simulink model "furutapendulumsim2"  (R2018a)
settings: Solver=VariableStepAuto  StartTime=0.0  StopTime=15  RelTol=1e-3
values from neighbouring files (symbols this model uses):
  A = [0,1,0,0 ... (first row only)    [furutapendulum.m]    (also in furutapendulum2.m = double(A); furutapendulum3.m = double(A); furutapendulum3_.m = double(A); furutapendulum4.m = double(A))
  B = [0 ... (first row only)    [furutapendulum.m]    (also in furutapendulum2.m = double(B); furutapendulum3.m = double(B); furutapendulum3_.m = double(B); furutapendulum4.m = double(B))
  length_base = 10e-3    (= 0.01)    [furutapendulum2.m]    (also in furutapendulum3.m; furutapendulum4.m)
  length_vert_cylinder = 200e-3    (= 0.2)    [furutapendulum2.m]    (also in furutapendulum3.m; furutapendulum4.m)
  m = 3.3e-3    (= 0.0033)    [furutapendulum2.m]    (also in furutapendulum3.m; furutapendulum4.m)
  radius_vert_cylinder = 10e-3    (= 0.01)    [furutapendulum2.m]    (also in furutapendulum3.m; furutapendulum4.m)
  s = tf('s')    [furutapendulum2.m]    (also in furutapendulum3.m; furutapendulum3_.m; furutapendulum4.m)
  Ts = 0.01    [furutapendulum2.m]    (also in furutapendulum3.m; furutapendulum4.m = 0.02)
undefined symbols (not defined in the file or in its folder): A1, A2, B1, B2, C1, C2, D1, D2, X, Y, Z
libraries: sm_lib x432, nesl_utility x54, cstblocks x17, aerolibanimutils x9, simulink x3
(part 2 of 13)

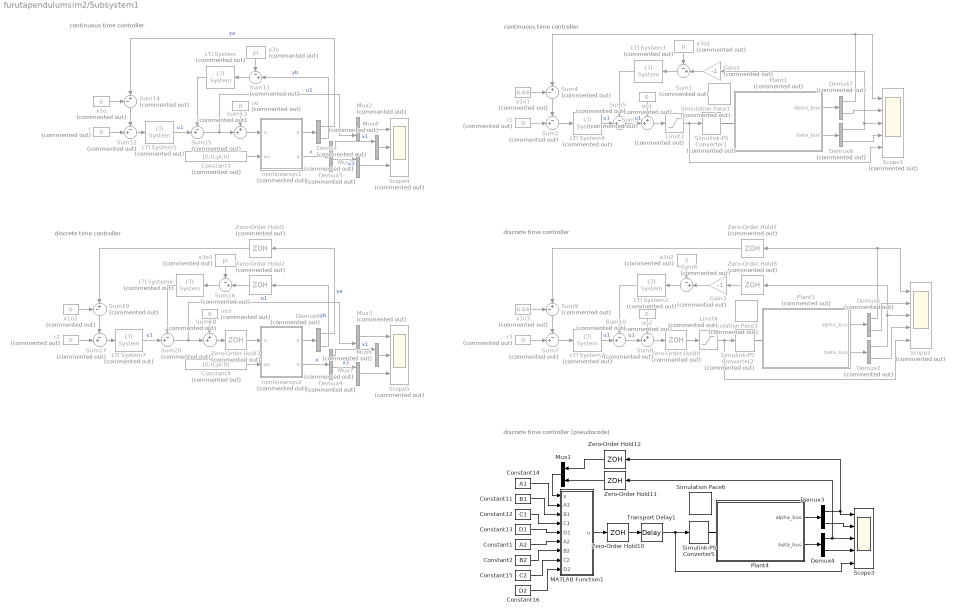
== system furutapendulumsim2/Subsystem1 ==
  note: continuous time controller
  note: discrete time controller (pseudocode)
  note: discrete time controller
  note: continuous time controller
  note: discrete time controller
  Constant1 : Constant  Value=A2
  Constant11 : Constant  Value=B1
  Constant12 : Constant  Value=C1
  Constant13 : Constant  Value=D1
  Constant14 : Constant  Value=A1
  Constant15 : Constant  Value=C2
  Constant16 : Constant  Value=D2
  Constant2 : Constant  Value=B2
  Constant3 : Constant  Commented=on  Value=[0;0;pi;0]
  Constant4 : Constant  Commented=on  Value=[0;0;pi;0]
  Demux{,1..2,6..8} (6 alike) : Demux  Commented=on  Outputs=2
  Demux3 : Demux  Outputs=2
  Demux4 : Demux  Outputs=2
  Demux5 : Demux  Commented=on
  Demux9 : Demux  Commented=on
  Gain2 : Gain  Commented=on  Gain=-1
  Gain3 : Gain  Commented=on  Gain=-1
  LTI System : cstblocks/LTI System  Commented=on  sys=Cc2  IC=[]
  LTI System1 : cstblocks/LTI System  Commented=on  sys=Cd2  IC=[]
  LTI System2 : cstblocks/LTI System  Commented=on  sys=Cd1  IC=[]
  LTI System3 : cstblocks/LTI System  Commented=on  sys=Cc2  IC=[]
  LTI System4 : cstblocks/LTI System  Commented=on  sys=Cc1  IC=[]
  LTI System5 : cstblocks/LTI System  Commented=on  sys=Cc1  IC=[]
  LTI System6 : cstblocks/LTI System  Commented=on  sys=Cd2  IC=[]
  LTI System7 : cstblocks/LTI System  Commented=on  sys=Cd1  IC=[]
  Limit3 : Saturate  Commented=on  UpperLimit=0.1e3  LowerLimit=-0.1e3
  Limit4 : Saturate  Commented=on  UpperLimit=0.1e3  LowerLimit=-0.1e3
  MATLAB Function1 : MATLAB Function  TreatAsAtomicUnit=on
  Mux1 : Mux  Inputs=2
  Mux{2..7} (6 alike) : Mux  Commented=on  Inputs=2
  Plant1 : Subsystem  Commented=on
      mask Display:
      | image('overall.JPG')
      | port_label('lconn',1,'torque');
      | port_label('output', 1, 'alpha_bus')
      | port_label('output', 2, 'beta_bus')
  Plant3 : Subsystem  Commented=on
      mask Display:
      | image('overall.JPG')
      | port_label('lconn',1,'torque');
      | port_label('output', 1, 'alpha_bus')
      | port_label('output', 2, 'beta_bus')
  Plant4 : Subsystem
      mask Display:
      | image('overall.JPG')
      | port_label('lconn',1,'torque');
      | port_label('output', 1, 'alpha_bus')
      | port_label('output', 2, 'beta_bus')
  Scope1 : Scope  Commented=on  NumInputPorts=5
  Scope2 : Scope  Commented=on  NumInputPorts=5
  Scope3 : Scope  NumInputPorts=5
  Scope4 : Scope  Commented=on  NumInputPorts=3
  Scope5 : Scope  Commented=on  NumInputPorts=3
  Simulation Pace1 : aerolibanimutils/Simulation Pace  Commented=on  SimulationPace=1  SleepMode=MATLAB Thread  OutputPaceError=off  SampleTime=1/30
      settings: AttributesFormatString=%<SimulationPace> sec/sec
  Simulation Pace3 : aerolibanimutils/Simulation Pace  Commented=on  SimulationPace=1  SleepMode=MATLAB Thread  OutputPaceError=off  SampleTime=1/30
      settings: AttributesFormatString=%<SimulationPace> sec/sec
  Simulation Pace6 : aerolibanimutils/Simulation Pace  SimulationPace=1  SleepMode=MATLAB Thread  OutputPaceError=off  SampleTime=1/30
      settings: AttributesFormatString=%<SimulationPace> sec/sec
  Simulink-PS Converter1 : nesl_utility/Simulink-PS Converter  Commented=on  PhysicalDomain=network_engine_domain  SubClassName=ps_input  LeftPortType=input  RightPortType=output  PseudoPeriodic=off  Frequencies=[]  NoiseDistribution=none  NoiseParameters=[]  Unit=N*mm  AffineConversion=off  FilteringAndDerivatives=zero  SimscapeFilterOrder=1  InputFilterTimeConstant=0.001  UdotUserProvided=1
  Simulink-PS Converter2 : nesl_utility/Simulink-PS Converter  Commented=on  PhysicalDomain=network_engine_domain  SubClassName=ps_input  LeftPortType=input  RightPortType=output  PseudoPeriodic=off  Frequencies=[]  NoiseDistribution=none  NoiseParameters=[]  Unit=N*mm  AffineConversion=off  FilteringAndDerivatives=zero  SimscapeFilterOrder=1  InputFilterTimeConstant=0.001  UdotUserProvided=1
  Simulink-PS Converter5 : nesl_utility/Simulink-PS Converter  PhysicalDomain=network_engine_domain  SubClassName=ps_input  LeftPortType=input  RightPortType=output  PseudoPeriodic=off  Frequencies=[]  NoiseDistribution=none  NoiseParameters=[]  Unit=N*mm  AffineConversion=off  FilteringAndDerivatives=zero  SimscapeFilterOrder=1  InputFilterTimeConstant=0.001  UdotUserProvided=1
  Sum{1..2,4..7,9..12,14..17,19..20} (16 alike) : Sum  Commented=on  Inputs=-+|
  Sum{3,8,13,18} (4 alike) : Sum  Commented=on  Inputs=++|
  Transport Delay1 : TransportDelay  DelayTime=Ts
  Zero-Order Hold{1..3,7..9} (6 alike) : ZeroOrderHold  Commented=on  SampleTime=Ts
  Zero-Order Hold10 : ZeroOrderHold  SampleTime=Ts
  Zero-Order Hold11 : ZeroOrderHold  SampleTime=Ts
  Zero-Order Hold12 : ZeroOrderHold  SampleTime=Ts
  nonlinearsys1 : Subsystem  Commented=on
  nonlinearsys2 : Subsystem  Commented=on
  r{,1..3} (4 alike) : Constant  Commented=on  Value=0
  uo{,1..3} (4 alike) : Constant  Commented=on  Value=0
  x1o : Constant  Commented=on  Value=0
  x1o1 : Constant  Commented=on  Value=6.64
  x1o2 : Constant  Commented=on  Value=0
  x1o3 : Constant  Commented=on  Value=6.64
  x3o : Constant  Commented=on  Value=pi
  x3o1 : Constant  Commented=on  Value=0
  x3o2 : Constant  Commented=on  Value=0
  x3o3 : Constant  Commented=on  Value=pi
  wires:
  Zero-Order Hold12/1 -> Mux1/1
  Demux1/1 -> Scope2/1, Zero-Order Hold7/1
  Mux1/1 -> MATLAB Function1/1(y)
  Zero-Order Hold11/1 -> Mux1/2
  Demux3/1 -> Scope3/1, Zero-Order Hold12/1
  MATLAB Function1/1(u) -> Zero-Order Hold10/1
  Zero-Order Hold7/1 -> Sum9/2
  Constant15/1 -> MATLAB Function1/8(C2)
  Transport Delay1/1 -> Scope3/5, Simulink-PS Converter5/1
  Demux2/2 -> Scope2/4
  Demux2/1 -> Scope2/3, Zero-Order Hold8/1
  Constant2/1 -> MATLAB Function1/7(B2)
  uo2/1 -> Sum8/1
  r3/1 -> Sum7/2
  Demux3/2 -> Scope3/2
  Sum9/1 -> Sum7/1
  Sum8/1 -> Zero-Order Hold9/1
  Constant1/1 -> MATLAB Function1/6(A2)
  Demux4/1 -> Scope3/3, Zero-Order Hold11/1
  x1o1/1 -> Sum4/1
  Demux4/2 -> Scope3/4
  Zero-Order Hold9/1 -> Limit4/1
  Constant14/1 -> MATLAB Function1/2(A1)
  Constant12/1 -> MATLAB Function1/4(C1)
  Constant11/1 -> MATLAB Function1/3(B1)
  Constant13/1 -> MATLAB Function1/5(D1)
  Sum10/1 -> Sum8/2  "u1"
  Plant3/1(alpha_bus) -> Demux1/1
  Plant4/1(alpha_bus) -> Demux3/1
  Demux7/2 -> Scope1/2
  Plant4/2(beta_bus) -> Demux4/1
  Sum7/1 -> LTI System2/1
  Demux1/2 -> Scope2/2
  Zero-Order Hold10/1 -> Transport Delay1/1
  LTI System2/1 -> Sum10/2  "u1"
  Limit3/1 -> Scope1/5, Simulink-PS Converter1/1
  Limit4/1 -> Scope2/5, Simulink-PS Converter2/1
  Gain2/1 -> Sum1/2
  Plant3/2(beta_bus) -> Demux2/1
  Plant1/2(beta_bus) -> Demux8/1
  Demux8/2 -> Scope1/4
  Sum1/1 -> LTI System3/1
  r1/1 -> Sum2/2
  uo1/1 -> Sum3/1
  Demux8/1 -> Gain2/1, Scope1/3
  Zero-Order Hold8/1 -> Gain3/1
  Plant1/1(alpha_bus) -> Demux7/1
  Demux7/1 -> Sum4/2, Scope1/1
  Sum4/1 -> Sum2/1
  Sum3/1 -> Limit3/1
  Sum5/1 -> Sum3/2  "u1"
  LTI System4/1 -> Sum5/2  "u1"
  x3o1/1 -> Sum1/1
  x1o3/1 -> Sum9/1
  Sum2/1 -> LTI System4/1
  Constant16/1 -> MATLAB Function1/9(D2)
  Sum13/1 -> nonlinearsys1/1("u ")
  Sum12/1 -> LTI System5/1
  Demux/2 -> Sum11/2  "yb"
  Sum11/1 -> LTI System/1
  nonlinearsys1/1(y) -> Demux/1
  nonlinearsys1/2(x) -> Demux5/1  "x"
  Mux4/1 -> Scope4/2
  x1o/1 -> Sum14/1
  Demux/1 -> Sum14/2  "ya"
  LTI System5/1 -> Sum15/2  "u1"
  Sum14/1 -> Sum12/1
  Mux5/1 -> Scope4/3
  x3o/1 -> Sum11/1
  uo/1 -> Sum13/1
  Constant3/1 -> nonlinearsys1/2(xo)
  Demux5/1 -> Mux4/1  "x1"
  Demux5/3 -> Mux5/1  "x3"
  Sum15/1 -> Sum13/2, Mux2/2  "u1"
  Mux2/1 -> Scope4/1
  r/1 -> Sum12/2
  LTI System3/1 -> Sum5/1
  x3o2/1 -> Sum6/1
  Gain3/1 -> Sum6/2
  Sum6/1 -> LTI System1/1
  LTI System1/1 -> Sum10/1
  LTI System/1 -> Sum15/1
  Mux6/1 -> Scope5/2
  x3o3/1 -> Sum16/1
  Mux7/1 -> Scope5/3
  LTI System7/1 -> Sum20/2  "u1"
  Sum19/1 -> Sum17/1
  x1o2/1 -> Sum19/1
  Demux9/1 -> Mux6/1  "x1"
  Demux6/1 -> Zero-Order Hold1/1  "ya"
  nonlinearsys2/1(y) -> Demux6/1
  Demux6/2 -> Zero-Order Hold2/1  "yb"
  r2/1 -> Sum17/2
  Mux3/1 -> Scope5/1
  uo3/1 -> Sum18/1
  Demux9/3 -> Mux7/1  "x3"
  Sum17/1 -> LTI System7/1
  Sum20/1 -> Sum18/2, Mux3/2  "u1"
  Sum16/1 -> LTI System6/1
  LTI System6/1 -> Sum20/1
  Constant4/1 -> nonlinearsys2/2(xo)
  nonlinearsys2/2(x) -> Demux9/1  "x"
  Zero-Order Hold1/1 -> Sum19/2
  Zero-Order Hold2/1 -> Sum16/2
  Sum18/1 -> Zero-Order Hold3/1
  Zero-Order Hold3/1 -> nonlinearsys2/1("u ")
  connections:
  Simulink-PS Converter5/RConn1 -- Plant4/LConn1
  Simulink-PS Converter1/RConn1 -- Plant1/LConn1
  Simulink-PS Converter2/RConn1 -- Plant3/LConn1

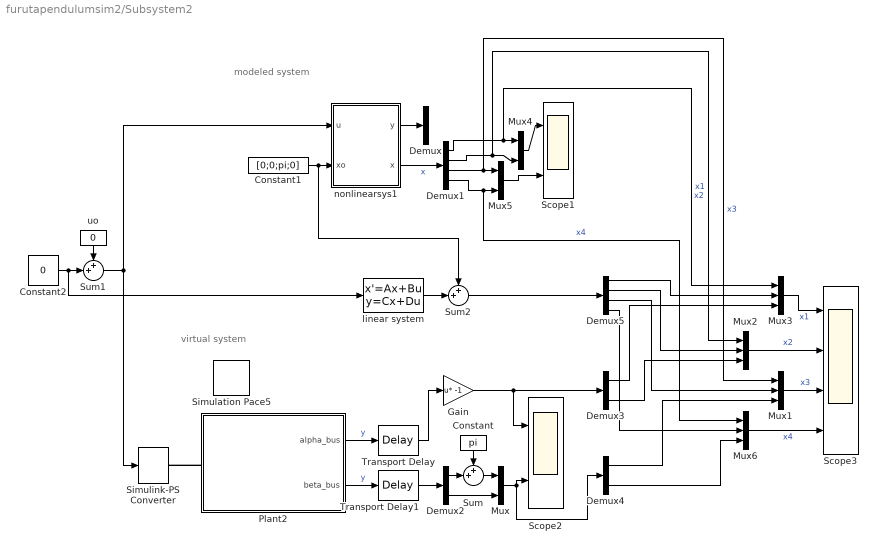
== system furutapendulumsim2/Subsystem2 ==
  note: modeled system
  note: virtual system
  Constant : Constant  Value=pi
  Constant1 : Constant  Value=[0;0;pi;0]
  Constant2 : Constant  Value=0
  Demux{,2..4} (4 alike) : Demux  Outputs=2
  Demux1 : Demux
  Demux5 : Demux
  Gain : Gain  Gain=-1  Multiplication=Matrix(u*K)
  Mux : Mux  Inputs=2
  Mux{1..3,6} (4 alike) : Mux  Inputs=3
  Mux4 : Mux  Inputs=2
  Mux5 : Mux  Inputs=2
  Plant2 : Subsystem
      mask Display:
      | image('overall.JPG')
      | port_label('lconn',1,'torque');
      | port_label('output', 1, 'alpha_bus')
      | port_label('output', 2, 'beta_bus')
  Scope1 : Scope  NumInputPorts=2
  Scope2 : Scope  NumInputPorts=2
  Scope3 : Scope  NumInputPorts=4
  Simulation Pace5 : aerolibanimutils/Simulation Pace  SimulationPace=1  SleepMode=MATLAB Thread  OutputPaceError=off  SampleTime=1/30
      settings: AttributesFormatString=%<SimulationPace> sec/sec
  Simulink-PS Converter : nesl_utility/Simulink-PS Converter  PhysicalDomain=network_engine_domain  SubClassName=ps_input  LeftPortType=input  RightPortType=output  PseudoPeriodic=off  Frequencies=[]  NoiseDistribution=none  NoiseParameters=[]  Unit=N*mm  AffineConversion=off  FilteringAndDerivatives=zero  SimscapeFilterOrder=1  InputFilterTimeConstant=0.001  UdotUserProvided=1
  Sum : Sum  Inputs=++|
  Sum1 : Sum  Inputs=++|
  Sum2 : Sum  Inputs=++|
  Transport Delay : TransportDelay  DelayTime=2
  Transport Delay1 : TransportDelay  DelayTime=2
  linear system : StateSpace  A=A  B=B  C=eye(4)  D=zeros(4,1)  InitialCondition=[0;0;0;0]
  nonlinearsys1 : Subsystem
  uo : Constant  Value=0
  wires:
  Demux2/2 -> Mux/2
  Demux1/3 -> Mux1/1, Mux5/1  "x3"
  Mux5/1 -> Scope1/2
  Mux4/1 -> Scope1/1
  Demux2/1 -> Sum/2
  Plant2/2(beta_bus) -> Transport Delay1/1  "y"
  Sum/1 -> Mux/1
  Constant/1 -> Sum/1
  Demux1/1 -> Mux3/1, Mux4/1  "x1"
  nonlinearsys1/1(y) -> Demux/1
  Constant1/1 -> Sum2/1, nonlinearsys1/2(xo)
  nonlinearsys1/2(x) -> Demux1/1  "x"
  Demux1/4 -> Mux6/1, Mux5/2  "x4"
  Demux1/2 -> Mux4/2, Mux2/1  "x2"
  Gain/1 -> Scope2/1, Demux3/1
  Plant2/1(alpha_bus) -> Transport Delay/1  "y"
  Mux3/1 -> Scope3/1  "x1"
  Mux2/1 -> Scope3/2  "x2"
  Mux1/1 -> Scope3/3  "x3"
  Mux6/1 -> Scope3/4  "x4"
  Demux3/1 -> Mux3/3
  Demux3/2 -> Mux2/3
  Demux4/1 -> Mux1/3
  Demux4/2 -> Mux6/3
  Transport Delay/1 -> Gain/1
  linear system/1 -> Sum2/2
  Sum2/1 -> Demux5/1
  Demux5/1 -> Mux3/2
  Demux5/2 -> Mux2/2
  Demux5/3 -> Mux1/2
  Demux5/4 -> Mux6/2
  uo/1 -> Sum1/1
  Constant2/1 -> linear system/1, Sum1/2
  Sum1/1 -> Simulink-PS Converter/1, nonlinearsys1/1("u ")
  Mux/1 -> Scope2/2, Demux4/1
  Transport Delay1/1 -> Demux2/1
  connections:
  Plant2/LConn1 -- Simulink-PS Converter/RConn1

== system furutapendulumsim2/nonlinearsys2 ==
  "u " : Inport
  xo : Inport  Port=2
  Integrator : Integrator  InitialConditionSource=external  InitialCondition=[0;0;0.5]
  MATLAB Function : MATLAB Function  TreatAsAtomicUnit=on
  MATLAB Function1 : MATLAB Function  TreatAsAtomicUnit=on
  y : Outport
  x : Outport  Port=2
  wires:
  xo/1 -> Integrator/2
  MATLAB Function/1(f) -> Integrator/1
  Integrator/1 -> x/1, MATLAB Function/1(x), MATLAB Function1/1(x)
  "u "/1 -> MATLAB Function1/2(u), MATLAB Function/2(u)
  MATLAB Function1/1(y) -> y/1

== system furutapendulumsim2/Controller1/Specific potential energy1 ==
  beta_bus : Inport
  Bus Selector2 : BusSelector  OutputSignals=beta
  Constant : Constant
  Sum : Sum  Inputs=|+-
  Trigonometric Function : Trigonometry  Operator=cos
  specific_energy : Outport
  wires:
  Constant/1 -> Sum/2
  Trigonometric Function/1 -> Sum/1
  Sum/1 -> specific_energy/1
  Bus Selector2/1 -> Trigonometric Function/1  "<beta>"
  beta_bus/1 -> Bus Selector2/1

== system furutapendulumsim2/Controller1/SwingUp_Control1 ==
  beta_bus : Inport
  normalized_energy : Inport  Port=2
  Bus Selector : BusSelector  OutputSignals=beta,dbeta
  Gain : Gain  Gain=Gain
  Product : Product
  Product1 : Product
  Sign : Signum
  Trigonometric Function : Trigonometry  Operator=cos
  ControlOutput : Outport
  wires:
  Product/1 -> Sign/1
  Trigonometric Function/1 -> Product/1
  Gain/1 -> ControlOutput/1
  Sign/1 -> Product1/2
  Product1/1 -> Gain/1
  normalized_energy/1 -> Product1/1
  beta_bus/1 -> Bus Selector/1
  Bus Selector/1 -> Trigonometric Function/1  "<beta>"
  Bus Selector/2 -> Product/2  "<dbeta>"

== system furutapendulumsim2/Plant1/h_39_axle_1_RIGID ==
  note: for visualisation only,
      | better isometric
  Solid : sm_lib/Body Elements/Solid  InertiaType=Custom  Mass=0.00052672018519800228  MassUnits=kg  CenterOfMass=[0 0 0]  CenterOfMassUnits=mm  MomentsOfInertia=[0.0012508560304239273 0.066771141817072402 0.066771141817072402]  MomentsOfInertiaUnits=kg*mm^2  ProductsOfInertia=[0 0 0]  ProductsOfInertiaUnits=kg*mm^2  DensityBased=on  Density=1000  DensityUnits=kg/(m^3)  DoExposeReferenceFrame=on  SerializedFrames=<Frames/>  GraphicType=FromGeometry  MarkerShape=Sphere  MarkerSize=10  MarkerSizeUnits=m  GraphicVisPropType=SimpleVisualProperties  GraphicDiffuseColor=[0.4 0.4 0.4]  GraphicSpecularColor=[0.5 0.5 0.5 1.0]  GraphicAmbientColor=[0.15 0.15 0.15 1.0]  GraphicEmissiveColor=[0.0 0.0 0.0 1.0]  GraphicShininess=75  GraphicOpacity=1  GeometryShape=FromFile  RectangleSize=[1 1]  RectangleSizeUnits=m  BrickDimensions=[1 1 1]  BrickDimensionUnits=m  CylinderRadius=1  CylinderRadiusUnits=m  CylinderLength=1  CylinderLengthUnits=m  SphereRadius=1  SphereRadiusUnits=m  EllipsoidRadii=[1 1 1]  EllipsoidRadiiUnits=m  ExtrusionCrossSection=[1 1; -1 1; -1 -1; 1 -1]  ExtrusionCrossSectionUnits=m  ExtrusionLength=1  ExtrusionLengthUnits=m  PolygonNumSides=3  PolygonOuterRadius=1  PolygonOuterRadiusUnits=m  ExtGeomFileType=STL  ExtGeomFileName=h_39_axle_Default_sldprt.STL  ExtGeomFileUnits=mm  RevolutionCrossSection=[1 1; 1 -1; 2 -1; 2 1]  RevolutionCrossSectionUnits=m  RevolutionExtent=Full  RevolutionAngle=180  RevolutionAngleUnits=deg
  Transform : sm_lib/Frames and Transforms/Rigid Transform  TranslationMethod=Cartesian  TranslationStandardOffset=0  TranslationLengthUnit=mm  TranslationStandardAxis=+Z  TranslationCartesianOffset=[19.5 1.2534832698893993 1.25543121904946712 ]  TranslationROffset=0  TranslationROffsetUnits=m  TranslationZOffset=0  TranslationZOffsetUnits=m  TranslationThetaOffset=0  TranslationThetaOffsetUnits=deg  RotationMethod=StandardAxis  RotationAngleUnits=rad  RotationStandardAxis=-Y  RotationAngle=pi/2  RotationArbitraryAxis=[0.70549464967288755 0.067487766045881178 -0.70549464967288456]  FollAlignAxisA=+X  BaseAlignAxisA=+Y  FollAlignAxisB=+Y  BaseAlignAxisB=+Z  RotationSequenceAxes=FollowerAxes  RotationSequence=XYX  RotationSequenceAngles=[0 0 0]  RotationSequenceAnglesUnits=deg  RotationMatrix=[1 0 0; 0 1 0; 0 0 1]
  Transform1 : sm_lib/Frames and Transforms/Rigid Transform  TranslationMethod=Cartesian  TranslationStandardOffset=0  TranslationLengthUnit=mm  TranslationStandardAxis=+Z  TranslationCartesianOffset=[0 0 19.5]  TranslationROffset=0  TranslationROffsetUnits=m  TranslationZOffset=0  TranslationZOffsetUnits=m  TranslationThetaOffset=0  TranslationThetaOffsetUnits=deg  RotationMethod=StandardAxis  RotationAngleUnits=rad  RotationStandardAxis=-Y  RotationAngle=pi/2  RotationArbitraryAxis=[0.70549464967288755 0.067487766045881178 -0.70549464967288456]  FollAlignAxisA=+X  BaseAlignAxisA=+Y  FollAlignAxisB=+Y  BaseAlignAxisB=+Z  RotationSequenceAxes=FollowerAxes  RotationSequence=XYX  RotationSequenceAngles=[0 0 0]  RotationSequenceAnglesUnits=deg  RotationMatrix=[1 0 0; 0 1 0; 0 0 1]
  Transform2 : sm_lib/Frames and Transforms/Rigid Transform  TranslationMethod=Cartesian  TranslationStandardOffset=0  TranslationLengthUnit=mm  TranslationStandardAxis=+Z  TranslationCartesianOffset=[0 0 19.5]  TranslationROffset=0  TranslationROffsetUnits=m  TranslationZOffset=0  TranslationZOffsetUnits=m  TranslationThetaOffset=0  TranslationThetaOffsetUnits=deg  RotationMethod=StandardAxis  RotationAngleUnits=rad  RotationStandardAxis=+Z  RotationAngle=pi  RotationArbitraryAxis=[0.70549464967288755 0.067487766045881178 -0.70549464967288456]  FollAlignAxisA=+X  BaseAlignAxisA=+Y  FollAlignAxisB=+Y  BaseAlignAxisB=+Z  RotationSequenceAxes=FollowerAxes  RotationSequence=XYX  RotationSequenceAngles=[0 0 0]  RotationSequenceAnglesUnits=deg  RotationMatrix=[1 0 0; 0 1 0; 0 0 1]
  B : PMIOPort  Side=Left
  F : PMIOPort  Port=2  Side=Right
  connections:
  Solid/RConn1 -- Transform1/RConn1 -- Transform/LConn1
  Transform/RConn1 -- F/RConn1
  Transform2/RConn1 -- Transform1/LConn1
  B/RConn1 -- Transform2/LConn1

== system furutapendulumsim2/Plant1/h_RIP_arm_v2_1_RIGID ==
  Transform : sm_lib/Frames and Transforms/Rigid Transform  TranslationMethod=Cartesian  TranslationStandardOffset=0  TranslationLengthUnit=mm  TranslationStandardAxis=+Z  TranslationCartesianOffset=[-2.3499999999999996 11.000000000000007 49.543413938003653]  TranslationROffset=0  TranslationROffsetUnits=m  TranslationZOffset=0  TranslationZOffsetUnits=m  TranslationThetaOffset=0  TranslationThetaOffsetUnits=deg  RotationMethod=ArbitraryAxis  RotationAngleUnits=rad  RotationStandardAxis=+Z  RotationAngle=2.0943951023931953  RotationArbitraryAxis=[0.57735026918962584 -0.57735026918962595 0.57735026918962562]  FollAlignAxisA=+X  BaseAlignAxisA=+Y  FollAlignAxisB=+Y  BaseAlignAxisB=+Z  RotationSequenceAxes=FollowerAxes  RotationSequence=XYX  RotationSequenceAngles=[0 0 0]  RotationSequenceAnglesUnits=deg  RotationMatrix=[1 0 0; 0 1 0; 0 0 1]
  Transform1 : sm_lib/Frames and Transforms/Rigid Transform  TranslationMethod=Cartesian  TranslationStandardOffset=0  TranslationLengthUnit=mm  TranslationStandardAxis=+Z  TranslationCartesianOffset=[52.337380238255371 20.27500000000154 24.811029445672951]  TranslationROffset=0  TranslationROffsetUnits=m  TranslationZOffset=0  TranslationZOffsetUnits=m  TranslationThetaOffset=0  TranslationThetaOffsetUnits=deg  RotationMethod=ArbitraryAxis  RotationAngleUnits=rad  RotationStandardAxis=+Z  RotationAngle=2.0943951023931953  RotationArbitraryAxis=[-0.57735026918962562 -0.57735026918962584 -0.57735026918962584]  FollAlignAxisA=+X  BaseAlignAxisA=+Y  FollAlignAxisB=+Y  BaseAlignAxisB=+Z  RotationSequenceAxes=FollowerAxes  RotationSequence=XYX  RotationSequenceAngles=[0 0 0]  RotationSequenceAnglesUnits=deg  RotationMatrix=[1 0 0; 0 1 0; 0 0 1]
  Transform2 : sm_lib/Frames and Transforms/Rigid Transform  TranslationMethod=Cartesian  TranslationStandardOffset=0  TranslationLengthUnit=mm  TranslationStandardAxis=+Z  TranslationCartesianOffset=[-2.3499999999999908 64.5 49.543413938003681]  TranslationROffset=0  TranslationROffsetUnits=m  TranslationZOffset=0  TranslationZOffsetUnits=m  TranslationThetaOffset=0  TranslationThetaOffsetUnits=deg  RotationMethod=ArbitraryAxis  RotationAngleUnits=rad  RotationStandardAxis=+Z  RotationAngle=1.5707963267948966  RotationArbitraryAxis=[0 0 1]  FollAlignAxisA=+X  BaseAlignAxisA=+Y  FollAlignAxisB=+Y  BaseAlignAxisB=+Z  RotationSequenceAxes=FollowerAxes  RotationSequence=XYX  RotationSequenceAngles=[0 0 0]  RotationSequenceAnglesUnits=deg  RotationMatrix=[1 0 0; 0 1 0; 0 0 1]
  Transform3 : sm_lib/Frames and Transforms/Rigid Transform  TranslationMethod=Cartesian  TranslationStandardOffset=0  TranslationLengthUnit=mm  TranslationStandardAxis=+Z  TranslationCartesianOffset=[-2.3499999999999908 56.699999999999996 49.543413938003681]  TranslationROffset=0  TranslationROffsetUnits=m  TranslationZOffset=0  TranslationZOffsetUnits=m  TranslationThetaOffset=0  TranslationThetaOffsetUnits=deg  RotationMethod=ArbitraryAxis  RotationAngleUnits=rad  RotationStandardAxis=+Z  RotationAngle=1.5707963267948966  RotationArbitraryAxis=[0 0 1]  FollAlignAxisA=+X  BaseAlignAxisA=+Y  FollAlignAxisB=+Y  BaseAlignAxisB=+Z  RotationSequenceAxes=FollowerAxes  RotationSequence=XYX  RotationSequenceAngles=[0 0 0]  RotationSequenceAnglesUnits=deg  RotationMatrix=[1 0 0; 0 1 0; 0 0 1]
  Transform4 : sm_lib/Frames and Transforms/Rigid Transform  TranslationMethod=Cartesian  TranslationStandardOffset=0  TranslationLengthUnit=mm  TranslationStandardAxis=+Z  TranslationCartesianOffset=[-2.3499999999999841 84.40000000000002 49.543413938003681]  TranslationROffset=0  TranslationROffsetUnits=m  TranslationZOffset=0  TranslationZOffsetUnits=m  TranslationThetaOffset=0  TranslationThetaOffsetUnits=deg  RotationMethod=ArbitraryAxis  RotationAngleUnits=rad  RotationStandardAxis=+Z  RotationAngle=1.5707963267948966  RotationArbitraryAxis=[0 0 1]  FollAlignAxisA=+X  BaseAlignAxisA=+Y  FollAlignAxisB=+Y  BaseAlignAxisB=+Z  RotationSequenceAxes=FollowerAxes  RotationSequence=XYX  RotationSequenceAngles=[0 0 0]  RotationSequenceAnglesUnits=deg  RotationMatrix=[1 0 0; 0 1 0; 0 0 1]
  Transform5 : sm_lib/Frames and Transforms/Rigid Transform  TranslationMethod=Cartesian  TranslationStandardOffset=0  TranslationLengthUnit=mm  TranslationStandardAxis=+Z  TranslationCartesianOffset=[-2.3499999999999979 16.900000000000002 49.543413938003681]  TranslationROffset=0  TranslationROffsetUnits=m  TranslationZOffset=0  TranslationZOffsetUnits=m  TranslationThetaOffset=0  TranslationThetaOffsetUnits=deg  RotationMethod=ArbitraryAxis  RotationAngleUnits=rad  RotationStandardAxis=+Z  RotationAngle=1.5707963267948966  RotationArbitraryAxis=[0 0 1]  FollAlignAxisA=+X  BaseAlignAxisA=+Y  FollAlignAxisB=+Y  BaseAlignAxisB=+Z  RotationSequenceAxes=FollowerAxes  RotationSequence=XYX  RotationSequenceAngles=[0 0 0]  RotationSequenceAnglesUnits=deg  RotationMatrix=[1 0 0; 0 1 0; 0 0 1]
  h_39_axle_1_RIGID : Subsystem
      mask Display: image('h_39_axle_1_RIGID.JPG')
  h_axle_asymmetric_1_RIGID : Subsystem
      mask Display: image('h_axle_asymmetric_1_RIGID.JPG')
  h_collar_1_RIGID : Subsystem
      mask Display: image('h_collar_1_RIGID.JPG')
  h_connector_straight_1_RIGID : Subsystem
      mask Display: image('h_connector_straight_1_RIGID.JPG')
  B : PMIOPort  Side=Left
  F : PMIOPort  Port=2  Side=Right
  connections:
  Transform/LConn1 -- Transform1/LConn1 -- Transform2/LConn1 -- Transform3/LConn1 -- Transform4/LConn1 -- Transform5/LConn1
  Transform1/RConn1 -- F/RConn1
  Transform2/RConn1 -- h_axle_asymmetric_1_RIGID/LConn1
  Transform3/RConn1 -- h_connector_straight_1_RIGID/LConn1
  Transform4/RConn1 -- h_39_axle_1_RIGID/LConn1
  Transform5/RConn1 -- h_collar_1_RIGID/LConn1
  Transform/RConn1 -- B/RConn1

== system furutapendulumsim2/Plant1/h_RIP_pendulum_1_RIGID ==
  Transform : sm_lib/Frames and Transforms/Rigid Transform  TranslationMethod=Cartesian  TranslationStandardOffset=0  TranslationLengthUnit=mm  TranslationStandardAxis=+Z  TranslationCartesianOffset=[-191.15757664014251 -77.513756526474566 -2.6766783819563784]  TranslationROffset=0  TranslationROffsetUnits=m  TranslationZOffset=0  TranslationZOffsetUnits=m  TranslationThetaOffset=0  TranslationThetaOffsetUnits=deg  RotationMethod=ArbitraryAxis  RotationAngleUnits=rad  RotationStandardAxis=+Z  RotationAngle=2.0943951023931988  RotationArbitraryAxis=[0.57735026918962673 -0.5773502691896244 0.57735026918962606]  FollAlignAxisA=+X  BaseAlignAxisA=+Y  FollAlignAxisB=+Y  BaseAlignAxisB=+Z  RotationSequenceAxes=FollowerAxes  RotationSequence=XYX  RotationSequenceAngles=[0 0 0]  RotationSequenceAnglesUnits=deg  RotationMatrix=[1 0 0; 0 1 0; 0 0 1]
  Transform1 : sm_lib/Frames and Transforms/Rigid Transform  TranslationMethod=Cartesian  TranslationStandardOffset=0  TranslationLengthUnit=mm  TranslationStandardAxis=+Z  TranslationCartesianOffset=[-136.47019640188407 -153.13875652647175 22.05570611037507]  TranslationROffset=0  TranslationROffsetUnits=m  TranslationZOffset=0  TranslationZOffsetUnits=m  TranslationThetaOffset=0  TranslationThetaOffsetUnits=deg  RotationMethod=ArbitraryAxis  RotationAngleUnits=rad  RotationStandardAxis=+Z  RotationAngle=1.5707963267948999  RotationArbitraryAxis=[0 0 1]  FollAlignAxisA=+X  BaseAlignAxisA=+Y  FollAlignAxisB=+Y  BaseAlignAxisB=+Z  RotationSequenceAxes=FollowerAxes  RotationSequence=XYX  RotationSequenceAngles=[0 0 0]  RotationSequenceAnglesUnits=deg  RotationMatrix=[1 0 0; 0 1 0; 0 0 1]
  Transform2 : sm_lib/Frames and Transforms/Rigid Transform  TranslationMethod=Cartesian  TranslationStandardOffset=0  TranslationLengthUnit=mm  TranslationStandardAxis=+Z  TranslationCartesianOffset=[-136.47019640188358 -165.03875652647181 128.15570611037563]  TranslationROffset=0  TranslationROffsetUnits=m  TranslationZOffset=0  TranslationZOffsetUnits=m  TranslationThetaOffset=0  TranslationThetaOffsetUnits=deg  RotationMethod=ArbitraryAxis  RotationAngleUnits=rad  RotationStandardAxis=+Z  RotationAngle=1.5707963267949003  RotationArbitraryAxis=[0 1 0]  FollAlignAxisA=+X  BaseAlignAxisA=+Y  FollAlignAxisB=+Y  BaseAlignAxisB=+Z  RotationSequenceAxes=FollowerAxes  RotationSequence=XYX  RotationSequenceAngles=[0 0 0]  RotationSequenceAnglesUnits=deg  RotationMatrix=[1 0 0; 0 1 0; 0 0 1]
  Transform3 : sm_lib/Frames and Transforms/Rigid Transform  TranslationMethod=Cartesian  TranslationStandardOffset=0  TranslationLengthUnit=mm  TranslationStandardAxis=+Z  TranslationCartesianOffset=[-136.47019640188373 -165.03875652647179 72.95570611037553]  TranslationROffset=0  TranslationROffsetUnits=m  TranslationZOffset=0  TranslationZOffsetUnits=m  TranslationThetaOffset=0  TranslationThetaOffsetUnits=deg  RotationMethod=ArbitraryAxis  RotationAngleUnits=rad  RotationStandardAxis=+Z  RotationAngle=1.5707963267949003  RotationArbitraryAxis=[0 1 0]  FollAlignAxisA=+X  BaseAlignAxisA=+Y  FollAlignAxisB=+Y  BaseAlignAxisB=+Z  RotationSequenceAxes=FollowerAxes  RotationSequence=XYX  RotationSequenceAngles=[0 0 0]  RotationSequenceAnglesUnits=deg  RotationMatrix=[1 0 0; 0 1 0; 0 0 1]
  Transform4 : sm_lib/Frames and Transforms/Rigid Transform  TranslationMethod=Cartesian  TranslationStandardOffset=0  TranslationLengthUnit=mm  TranslationStandardAxis=+Z  TranslationCartesianOffset=[-136.47019640188347 -165.03875652647181 159.85570611037573]  TranslationROffset=0  TranslationROffsetUnits=m  TranslationZOffset=0  TranslationZOffsetUnits=m  TranslationThetaOffset=0  TranslationThetaOffsetUnits=deg  RotationMethod=ArbitraryAxis  RotationAngleUnits=rad  RotationStandardAxis=+Z  RotationAngle=1.5707963267949003  RotationArbitraryAxis=[0 1 0]  FollAlignAxisA=+X  BaseAlignAxisA=+Y  FollAlignAxisB=+Y  BaseAlignAxisB=+Z  RotationSequenceAxes=FollowerAxes  RotationSequence=XYX  RotationSequenceAngles=[0 0 0]  RotationSequenceAnglesUnits=deg  RotationMatrix=[1 0 0; 0 1 0; 0 0 1]
  Transform5 : sm_lib/Frames and Transforms/Rigid Transform  TranslationMethod=Cartesian  TranslationStandardOffset=0  TranslationLengthUnit=mm  TranslationStandardAxis=+Z  TranslationCartesianOffset=[-136.47019640188347 -165.03875652647181 159.85570611037573]  TranslationROffset=0  TranslationROffsetUnits=m  TranslationZOffset=0  TranslationZOffsetUnits=m  TranslationThetaOffset=0  TranslationThetaOffsetUnits=deg  RotationMethod=ArbitraryAxis  RotationAngleUnits=rad  RotationStandardAxis=+Z  RotationAngle=1.5707963267949003  RotationArbitraryAxis=[0 1 0]  FollAlignAxisA=+X  BaseAlignAxisA=+Y  FollAlignAxisB=+Y  BaseAlignAxisB=+Z  RotationSequenceAxes=FollowerAxes  RotationSequence=XYX  RotationSequenceAngles=[0 0 0]  RotationSequenceAnglesUnits=deg  RotationMatrix=[1 0 0; 0 1 0; 0 0 1]
  Transform6 : sm_lib/Frames and Transforms/Rigid Transform  TranslationMethod=Cartesian  TranslationStandardOffset=0  TranslationLengthUnit=mm  TranslationStandardAxis=+Z  TranslationCartesianOffset=[-94.97019640188347/2 -0 0]  TranslationROffset=0  TranslationROffsetUnits=m  TranslationZOffset=0  TranslationZOffsetUnits=m  TranslationThetaOffset=0  TranslationThetaOffsetUnits=deg  RotationMethod=None  RotationAngleUnits=rad  RotationStandardAxis=+Z  RotationAngle=1.5707963267949003  RotationArbitraryAxis=[0 1 0]  FollAlignAxisA=+X  BaseAlignAxisA=+Y  FollAlignAxisB=+Y  BaseAlignAxisB=+Z  RotationSequenceAxes=FollowerAxes  RotationSequence=XYX  RotationSequenceAngles=[0 0 0]  RotationSequenceAnglesUnits=deg  RotationMatrix=[1 0 0; 0 1 0; 0 0 1]
  h_10_axle_1_RIGID : Subsystem
      mask Display: image('h_39_axle_1_RIGID.JPG')
  h_79_axle_1_RIGID : Subsystem
      mask Display: image('h_39_axle_1_RIGID.JPG')
  h_connector_right_angle_1_RIGID : Subsystem
      mask Display: image('connector_right_angle_1_RIGID.JPG');
  h_connector_straight_1_RIGID : Subsystem
      mask Display: image('h_connector_straight_1_RIGID.JPG')
  h_connector_straight_1_RIGID1 : Subsystem
      mask Display: image('h_connector_straight_1_RIGID.JPG')
  F : PMIOPort  Side=Left
  connections:
  Transform/LConn1 -- Transform1/LConn1 -- Transform2/LConn1 -- Transform3/LConn1 -- Transform5/LConn1 -- Transform4/LConn1
  Transform/RConn1 -- F/RConn1
  Transform1/RConn1 -- h_connector_right_angle_1_RIGID/LConn1
  Transform2/RConn1 -- h_connector_straight_1_RIGID/LConn1
  Transform3/RConn1 -- h_10_axle_1_RIGID/LConn1
  Transform4/RConn1 -- h_79_axle_1_RIGID/LConn1
  Transform5/RConn1 -- Transform6/LConn1
  Transform6/RConn1 -- h_connector_straight_1_RIGID1/LConn1

== system furutapendulumsim2/Plant1/h_encoderaxles_1_RIGID ==
  Design_Correction : sm_lib/Frames and Transforms/Rigid Transform  TranslationMethod=None  TranslationStandardOffset=0  TranslationLengthUnit=mm  TranslationStandardAxis=+Z  TranslationCartesianOffset=[24.508089637866071 17.711031392187333 8.5401255470870616]  TranslationROffset=0  TranslationROffsetUnits=m  TranslationZOffset=0  TranslationZOffsetUnits=m  TranslationThetaOffset=0  TranslationThetaOffsetUnits=deg  RotationMethod=ArbitraryAxis  RotationAngleUnits=rad  RotationStandardAxis=+Z  RotationAngle=-pi/2-3.0420956054916015  RotationArbitraryAxis=[-0 0 -1]  FollAlignAxisA=+X  BaseAlignAxisA=+Y  FollAlignAxisB=+Y  BaseAlignAxisB=+Z  RotationSequenceAxes=FollowerAxes  RotationSequence=XYX  RotationSequenceAngles=[0 0 0]  RotationSequenceAnglesUnits=deg  RotationMatrix=[1 0 0; 0 1 0; 0 0 1]
  Transform : sm_lib/Frames and Transforms/Rigid Transform  TranslationMethod=Cartesian  TranslationStandardOffset=0  TranslationLengthUnit=mm  TranslationStandardAxis=+Z  TranslationCartesianOffset=[24.508089637866071 17.711031392187333 8.5401255470870616]  TranslationROffset=0  TranslationROffsetUnits=m  TranslationZOffset=0  TranslationZOffsetUnits=m  TranslationThetaOffset=0  TranslationThetaOffsetUnits=deg  RotationMethod=ArbitraryAxis  RotationAngleUnits=rad  RotationStandardAxis=+Z  RotationAngle=3.0420956054916015  RotationArbitraryAxis=[-1 1.5754106539324166e-16 -3.1641356201816969e-15]  FollAlignAxisA=+X  BaseAlignAxisA=+Y  FollAlignAxisB=+Y  BaseAlignAxisB=+Z  RotationSequenceAxes=FollowerAxes  RotationSequence=XYX  RotationSequenceAngles=[0 0 0]  RotationSequenceAnglesUnits=deg  RotationMatrix=[1 0 0; 0 1 0; 0 0 1]
  Transform1 : sm_lib/Frames and Transforms/Rigid Transform  TranslationMethod=Cartesian  TranslationStandardOffset=0  TranslationLengthUnit=mm  TranslationStandardAxis=+Z  TranslationCartesianOffset=[13.983089637865053 16.866870285554842 29.580332105627452]  TranslationROffset=0  TranslationROffsetUnits=m  TranslationZOffset=0  TranslationZOffsetUnits=m  TranslationThetaOffset=0  TranslationThetaOffsetUnits=deg  RotationMethod=ArbitraryAxis  RotationAngleUnits=rad  RotationStandardAxis=+Z  RotationAngle=2.0943951023931975  RotationArbitraryAxis=[-0.57735026918962429 -0.57735026918962629 0.57735026918962662]  FollAlignAxisA=+X  BaseAlignAxisA=+Y  FollAlignAxisB=+Y  BaseAlignAxisB=+Z  RotationSequenceAxes=FollowerAxes  RotationSequence=XYX  RotationSequenceAngles=[0 0 0]  RotationSequenceAnglesUnits=deg  RotationMatrix=[1 0 0; 0 1 0; 0 0 1]
  Transform2 : sm_lib/Frames and Transforms/Rigid Transform  TranslationMethod=Cartesian  TranslationStandardOffset=0  TranslationLengthUnit=mm  TranslationStandardAxis=+Z  TranslationCartesianOffset=[3.9830896378650893 0.057027133562839033 -3.3724154764092837]  TranslationROffset=0  TranslationROffsetUnits=m  TranslationZOffset=0  TranslationZOffsetUnits=m  TranslationThetaOffset=0  TranslationThetaOffsetUnits=deg  RotationMethod=ArbitraryAxis  RotationAngleUnits=rad  RotationStandardAxis=+Z  RotationAngle=2.152761273624384  RotationArbitraryAxis=[0.59556683818013412 0.53907354092019244 0.59556683818013556]  FollAlignAxisA=+X  BaseAlignAxisA=+Y  FollAlignAxisB=+Y  BaseAlignAxisB=+Z  RotationSequenceAxes=FollowerAxes  RotationSequence=XYX  RotationSequenceAngles=[0 0 0]  RotationSequenceAnglesUnits=deg  RotationMatrix=[1 0 0; 0 1 0; 0 0 1]
  Transform3 : sm_lib/Frames and Transforms/Rigid Transform  TranslationMethod=Cartesian  TranslationStandardOffset=0  TranslationLengthUnit=mm  TranslationStandardAxis=+Z  TranslationCartesianOffset=[88.258089637865453 17.276122100546619 25.480708592190474]  TranslationROffset=0  TranslationROffsetUnits=m  TranslationZOffset=0  TranslationZOffsetUnits=m  TranslationThetaOffset=0  TranslationThetaOffsetUnits=deg  RotationMethod=ArbitraryAxis  RotationAngleUnits=rad  RotationStandardAxis=+Z  RotationAngle=3.071252132689227  RotationArbitraryAxis=[-0.70666895787164763 -0.70666895787165263 -0.03518476888075537]  FollAlignAxisA=+X  BaseAlignAxisA=+Y  FollAlignAxisB=+Y  BaseAlignAxisB=+Z  RotationSequenceAxes=FollowerAxes  RotationSequence=XYX  RotationSequenceAngles=[0 0 0]  RotationSequenceAnglesUnits=deg  RotationMatrix=[1 0 0; 0 1 0; 0 0 1]
  Transform4 : sm_lib/Frames and Transforms/Rigid Transform  TranslationMethod=Cartesian  TranslationStandardOffset=0  TranslationLengthUnit=mm  TranslationStandardAxis=+Z  TranslationCartesianOffset=[23.258089637866103 19.749512924159973 0.70385774641775622]  TranslationROffset=0  TranslationROffsetUnits=m  TranslationZOffset=0  TranslationZOffsetUnits=m  TranslationThetaOffset=0  TranslationThetaOffsetUnits=deg  RotationMethod=ArbitraryAxis  RotationAngleUnits=rad  RotationStandardAxis=+Z  RotationAngle=3.0712521326892568  RotationArbitraryAxis=[-0.70666895787165274 -0.035184768880752892 0.70666895787164763]  FollAlignAxisA=+X  BaseAlignAxisA=+Y  FollAlignAxisB=+Y  BaseAlignAxisB=+Z  RotationSequenceAxes=FollowerAxes  RotationSequence=XYX  RotationSequenceAngles=[0 0 0]  RotationSequenceAnglesUnits=deg  RotationMatrix=[1 0 0; 0 1 0; 0 0 1]
  Transform5 : sm_lib/Frames and Transforms/Rigid Transform  TranslationMethod=Cartesian  TranslationStandardOffset=0  TranslationLengthUnit=mm  TranslationStandardAxis=+Z  TranslationCartesianOffset=[47.083089637865008 15.289827696924307 45.378138349144159]  TranslationROffset=0  TranslationROffsetUnits=m  TranslationZOffset=0  TranslationZOffsetUnits=m  TranslationThetaOffset=0  TranslationThetaOffsetUnits=deg  RotationMethod=ArbitraryAxis  RotationAngleUnits=rad  RotationStandardAxis=+Z  RotationAngle=3.1415926535897882  RotationArbitraryAxis=[2.3430246690306488e-15 -0.67106893654685129 -0.74139495709228975]  FollAlignAxisA=+X  BaseAlignAxisA=+Y  FollAlignAxisB=+Y  BaseAlignAxisB=+Z  RotationSequenceAxes=FollowerAxes  RotationSequence=XYX  RotationSequenceAngles=[0 0 0]  RotationSequenceAnglesUnits=deg  RotationMatrix=[1 0 0; 0 1 0; 0 0 1]
  Transform6 : sm_lib/Frames and Transforms/Rigid Transform  TranslationMethod=Cartesian  TranslationStandardOffset=0  TranslationLengthUnit=mm  TranslationStandardAxis=+Z  TranslationCartesianOffset=[47.083089637865342 1.032411190979611 28.000963750391605]  TranslationROffset=0  TranslationROffsetUnits=m  TranslationZOffset=0  TranslationZOffsetUnits=m  TranslationThetaOffset=0  TranslationThetaOffsetUnits=deg  RotationMethod=ArbitraryAxis  RotationAngleUnits=rad  RotationStandardAxis=+Z  RotationAngle=3.1415926535897882  RotationArbitraryAxis=[2.3430246690306472e-15 -0.67106893654685129 -0.74139495709228975]  FollAlignAxisA=+X  BaseAlignAxisA=+Y  FollAlignAxisB=+Y  BaseAlignAxisB=+Z  RotationSequenceAxes=FollowerAxes  RotationSequence=XYX  RotationSequenceAngles=[0 0 0]  RotationSequenceAnglesUnits=deg  RotationMatrix=[1 0 0; 0 1 0; 0 0 1]
  Transform7 : sm_lib/Frames and Transforms/Rigid Transform  TranslationMethod=Cartesian  TranslationStandardOffset=0  TranslationLengthUnit=mm  TranslationStandardAxis=+Z  TranslationCartesianOffset=[47.083089637864894 32.667002295676816 31.120721843199458]  TranslationROffset=0  TranslationROffsetUnits=m  TranslationZOffset=0  TranslationZOffsetUnits=m  TranslationThetaOffset=0  TranslationThetaOffsetUnits=deg  RotationMethod=ArbitraryAxis  RotationAngleUnits=rad  RotationStandardAxis=+Z  RotationAngle=3.1415926535897882  RotationArbitraryAxis=[2.3430246690306472e-15 -0.67106893654685129 -0.74139495709228975]  FollAlignAxisA=+X  BaseAlignAxisA=+Y  FollAlignAxisB=+Y  BaseAlignAxisB=+Z  RotationSequenceAxes=FollowerAxes  RotationSequence=XYX  RotationSequenceAngles=[0 0 0]  RotationSequenceAnglesUnits=deg  RotationMatrix=[1 0 0; 0 1 0; 0 0 1]
  connector_right_angle_1_RIGID : Subsystem
      mask Display: image('connector_right_angle_1_RIGID.JPG');
  glidewheel_encoder_2_RIGID : Subsystem
      mask Display: image('glidewheel_encoder_2_RIGID.JPG');
  h_triangle_1_RIGID : Subsystem
      mask Display: image('h_triangle_1_RIGID.JPG')
  x86_axle_4_RIGID : Subsystem
      mask Display: image('x86_axle_4_RIGID.JPG')
  x86_axle_5_RIGID : Subsystem
      mask Display: image('x86_axle_4_RIGID.JPG')
  x86_axle_6_RIGID : Subsystem
      mask Display: image('x86_axle_4_RIGID.JPG')
  B : PMIOPort  Side=Left
  F : PMIOPort  Port=2  Side=Right
  connections:
  Design_Correction/RConn1 -- F/RConn1
  Transform2/RConn1 -- glidewheel_encoder_2_RIGID/LConn1
  Transform3/RConn1 -- h_triangle_1_RIGID/LConn1
  Transform4/RConn1 -- connector_right_angle_1_RIGID/LConn1
  Transform5/RConn1 -- x86_axle_4_RIGID/LConn1
  Transform6/RConn1 -- x86_axle_5_RIGID/LConn1
  Transform7/RConn1 -- x86_axle_6_RIGID/LConn1
  Transform/RConn1 -- B/RConn1
  Transform/LConn1 -- Transform7/LConn1 -- Transform6/LConn1 -- Transform5/LConn1 -- Transform4/LConn1 -- Transform3/LConn1 -- Transform2/LConn1 -- Transform1/LConn1
  Transform1/RConn1 -- Design_Correction/LConn1

== system furutapendulumsim2/Plant2/h_39_axle_1_RIGID ==
  note: for visualisation only,
      | better isometric
  Solid : sm_lib/Body Elements/Solid  InertiaType=Custom  Mass=0.00052672018519800228  MassUnits=kg  CenterOfMass=[0 0 0]  CenterOfMassUnits=mm  MomentsOfInertia=[0.0012508560304239273 0.066771141817072402 0.066771141817072402]  MomentsOfInertiaUnits=kg*mm^2  ProductsOfInertia=[0 0 0]  ProductsOfInertiaUnits=kg*mm^2  DensityBased=on  Density=1000  DensityUnits=kg/(m^3)  DoExposeReferenceFrame=on  SerializedFrames=<Frames/>  GraphicType=FromGeometry  MarkerShape=Sphere  MarkerSize=10  MarkerSizeUnits=m  GraphicVisPropType=SimpleVisualProperties  GraphicDiffuseColor=[0.4 0.4 0.4]  GraphicSpecularColor=[0.5 0.5 0.5 1.0]  GraphicAmbientColor=[0.15 0.15 0.15 1.0]  GraphicEmissiveColor=[0.0 0.0 0.0 1.0]  GraphicShininess=75  GraphicOpacity=1  GeometryShape=FromFile  RectangleSize=[1 1]  RectangleSizeUnits=m  BrickDimensions=[1 1 1]  BrickDimensionUnits=m  CylinderRadius=1  CylinderRadiusUnits=m  CylinderLength=1  CylinderLengthUnits=m  SphereRadius=1  SphereRadiusUnits=m  EllipsoidRadii=[1 1 1]  EllipsoidRadiiUnits=m  ExtrusionCrossSection=[1 1; -1 1; -1 -1; 1 -1]  ExtrusionCrossSectionUnits=m  ExtrusionLength=1  ExtrusionLengthUnits=m  PolygonNumSides=3  PolygonOuterRadius=1  PolygonOuterRadiusUnits=m  ExtGeomFileType=STL  ExtGeomFileName=h_39_axle_Default_sldprt.STL  ExtGeomFileUnits=mm  RevolutionCrossSection=[1 1; 1 -1; 2 -1; 2 1]  RevolutionCrossSectionUnits=m  RevolutionExtent=Full  RevolutionAngle=180  RevolutionAngleUnits=deg
  Transform : sm_lib/Frames and Transforms/Rigid Transform  TranslationMethod=Cartesian  TranslationStandardOffset=0  TranslationLengthUnit=mm  TranslationStandardAxis=+Z  TranslationCartesianOffset=[19.5 1.2534832698893993 1.25543121904946712 ]  TranslationROffset=0  TranslationROffsetUnits=m  TranslationZOffset=0  TranslationZOffsetUnits=m  TranslationThetaOffset=0  TranslationThetaOffsetUnits=deg  RotationMethod=StandardAxis  RotationAngleUnits=rad  RotationStandardAxis=-Y  RotationAngle=pi/2  RotationArbitraryAxis=[0.70549464967288755 0.067487766045881178 -0.70549464967288456]  FollAlignAxisA=+X  BaseAlignAxisA=+Y  FollAlignAxisB=+Y  BaseAlignAxisB=+Z  RotationSequenceAxes=FollowerAxes  RotationSequence=XYX  RotationSequenceAngles=[0 0 0]  RotationSequenceAnglesUnits=deg  RotationMatrix=[1 0 0; 0 1 0; 0 0 1]
  Transform1 : sm_lib/Frames and Transforms/Rigid Transform  TranslationMethod=Cartesian  TranslationStandardOffset=0  TranslationLengthUnit=mm  TranslationStandardAxis=+Z  TranslationCartesianOffset=[0 0 19.5]  TranslationROffset=0  TranslationROffsetUnits=m  TranslationZOffset=0  TranslationZOffsetUnits=m  TranslationThetaOffset=0  TranslationThetaOffsetUnits=deg  RotationMethod=StandardAxis  RotationAngleUnits=rad  RotationStandardAxis=-Y  RotationAngle=pi/2  RotationArbitraryAxis=[0.70549464967288755 0.067487766045881178 -0.70549464967288456]  FollAlignAxisA=+X  BaseAlignAxisA=+Y  FollAlignAxisB=+Y  BaseAlignAxisB=+Z  RotationSequenceAxes=FollowerAxes  RotationSequence=XYX  RotationSequenceAngles=[0 0 0]  RotationSequenceAnglesUnits=deg  RotationMatrix=[1 0 0; 0 1 0; 0 0 1]
  Transform2 : sm_lib/Frames and Transforms/Rigid Transform  TranslationMethod=Cartesian  TranslationStandardOffset=0  TranslationLengthUnit=mm  TranslationStandardAxis=+Z  TranslationCartesianOffset=[0 0 19.5]  TranslationROffset=0  TranslationROffsetUnits=m  TranslationZOffset=0  TranslationZOffsetUnits=m  TranslationThetaOffset=0  TranslationThetaOffsetUnits=deg  RotationMethod=StandardAxis  RotationAngleUnits=rad  RotationStandardAxis=+Z  RotationAngle=pi  RotationArbitraryAxis=[0.70549464967288755 0.067487766045881178 -0.70549464967288456]  FollAlignAxisA=+X  BaseAlignAxisA=+Y  FollAlignAxisB=+Y  BaseAlignAxisB=+Z  RotationSequenceAxes=FollowerAxes  RotationSequence=XYX  RotationSequenceAngles=[0 0 0]  RotationSequenceAnglesUnits=deg  RotationMatrix=[1 0 0; 0 1 0; 0 0 1]
  B : PMIOPort  Side=Left
  F : PMIOPort  Port=2  Side=Right
  connections:
  Solid/RConn1 -- Transform1/RConn1 -- Transform/LConn1
  Transform/RConn1 -- F/RConn1
  Transform2/RConn1 -- Transform1/LConn1
  B/RConn1 -- Transform2/LConn1

== system furutapendulumsim2/Plant2/h_RIP_arm_v2_1_RIGID ==
  Transform : sm_lib/Frames and Transforms/Rigid Transform  TranslationMethod=Cartesian  TranslationStandardOffset=0  TranslationLengthUnit=mm  TranslationStandardAxis=+Z  TranslationCartesianOffset=[-2.3499999999999996 11.000000000000007 49.543413938003653]  TranslationROffset=0  TranslationROffsetUnits=m  TranslationZOffset=0  TranslationZOffsetUnits=m  TranslationThetaOffset=0  TranslationThetaOffsetUnits=deg  RotationMethod=ArbitraryAxis  RotationAngleUnits=rad  RotationStandardAxis=+Z  RotationAngle=2.0943951023931953  RotationArbitraryAxis=[0.57735026918962584 -0.57735026918962595 0.57735026918962562]  FollAlignAxisA=+X  BaseAlignAxisA=+Y  FollAlignAxisB=+Y  BaseAlignAxisB=+Z  RotationSequenceAxes=FollowerAxes  RotationSequence=XYX  RotationSequenceAngles=[0 0 0]  RotationSequenceAnglesUnits=deg  RotationMatrix=[1 0 0; 0 1 0; 0 0 1]
  Transform1 : sm_lib/Frames and Transforms/Rigid Transform  TranslationMethod=Cartesian  TranslationStandardOffset=0  TranslationLengthUnit=mm  TranslationStandardAxis=+Z  TranslationCartesianOffset=[52.337380238255371 20.27500000000154 24.811029445672951]  TranslationROffset=0  TranslationROffsetUnits=m  TranslationZOffset=0  TranslationZOffsetUnits=m  TranslationThetaOffset=0  TranslationThetaOffsetUnits=deg  RotationMethod=ArbitraryAxis  RotationAngleUnits=rad  RotationStandardAxis=+Z  RotationAngle=2.0943951023931953  RotationArbitraryAxis=[-0.57735026918962562 -0.57735026918962584 -0.57735026918962584]  FollAlignAxisA=+X  BaseAlignAxisA=+Y  FollAlignAxisB=+Y  BaseAlignAxisB=+Z  RotationSequenceAxes=FollowerAxes  RotationSequence=XYX  RotationSequenceAngles=[0 0 0]  RotationSequenceAnglesUnits=deg  RotationMatrix=[1 0 0; 0 1 0; 0 0 1]
  Transform2 : sm_lib/Frames and Transforms/Rigid Transform  TranslationMethod=Cartesian  TranslationStandardOffset=0  TranslationLengthUnit=mm  TranslationStandardAxis=+Z  TranslationCartesianOffset=[-2.3499999999999908 64.5 49.543413938003681]  TranslationROffset=0  TranslationROffsetUnits=m  TranslationZOffset=0  TranslationZOffsetUnits=m  TranslationThetaOffset=0  TranslationThetaOffsetUnits=deg  RotationMethod=ArbitraryAxis  RotationAngleUnits=rad  RotationStandardAxis=+Z  RotationAngle=1.5707963267948966  RotationArbitraryAxis=[0 0 1]  FollAlignAxisA=+X  BaseAlignAxisA=+Y  FollAlignAxisB=+Y  BaseAlignAxisB=+Z  RotationSequenceAxes=FollowerAxes  RotationSequence=XYX  RotationSequenceAngles=[0 0 0]  RotationSequenceAnglesUnits=deg  RotationMatrix=[1 0 0; 0 1 0; 0 0 1]
  Transform3 : sm_lib/Frames and Transforms/Rigid Transform  TranslationMethod=Cartesian  TranslationStandardOffset=0  TranslationLengthUnit=mm  TranslationStandardAxis=+Z  TranslationCartesianOffset=[-2.3499999999999908 56.699999999999996 49.543413938003681]  TranslationROffset=0  TranslationROffsetUnits=m  TranslationZOffset=0  TranslationZOffsetUnits=m  TranslationThetaOffset=0  TranslationThetaOffsetUnits=deg  RotationMethod=ArbitraryAxis  RotationAngleUnits=rad  RotationStandardAxis=+Z  RotationAngle=1.5707963267948966  RotationArbitraryAxis=[0 0 1]  FollAlignAxisA=+X  BaseAlignAxisA=+Y  FollAlignAxisB=+Y  BaseAlignAxisB=+Z  RotationSequenceAxes=FollowerAxes  RotationSequence=XYX  RotationSequenceAngles=[0 0 0]  RotationSequenceAnglesUnits=deg  RotationMatrix=[1 0 0; 0 1 0; 0 0 1]
  Transform4 : sm_lib/Frames and Transforms/Rigid Transform  TranslationMethod=Cartesian  TranslationStandardOffset=0  TranslationLengthUnit=mm  TranslationStandardAxis=+Z  TranslationCartesianOffset=[-2.3499999999999841 84.40000000000002 49.543413938003681]  TranslationROffset=0  TranslationROffsetUnits=m  TranslationZOffset=0  TranslationZOffsetUnits=m  TranslationThetaOffset=0  TranslationThetaOffsetUnits=deg  RotationMethod=ArbitraryAxis  RotationAngleUnits=rad  RotationStandardAxis=+Z  RotationAngle=1.5707963267948966  RotationArbitraryAxis=[0 0 1]  FollAlignAxisA=+X  BaseAlignAxisA=+Y  FollAlignAxisB=+Y  BaseAlignAxisB=+Z  RotationSequenceAxes=FollowerAxes  RotationSequence=XYX  RotationSequenceAngles=[0 0 0]  RotationSequenceAnglesUnits=deg  RotationMatrix=[1 0 0; 0 1 0; 0 0 1]
  Transform5 : sm_lib/Frames and Transforms/Rigid Transform  TranslationMethod=Cartesian  TranslationStandardOffset=0  TranslationLengthUnit=mm  TranslationStandardAxis=+Z  TranslationCartesianOffset=[-2.3499999999999979 16.900000000000002 49.543413938003681]  TranslationROffset=0  TranslationROffsetUnits=m  TranslationZOffset=0  TranslationZOffsetUnits=m  TranslationThetaOffset=0  TranslationThetaOffsetUnits=deg  RotationMethod=ArbitraryAxis  RotationAngleUnits=rad  RotationStandardAxis=+Z  RotationAngle=1.5707963267948966  RotationArbitraryAxis=[0 0 1]  FollAlignAxisA=+X  BaseAlignAxisA=+Y  FollAlignAxisB=+Y  BaseAlignAxisB=+Z  RotationSequenceAxes=FollowerAxes  RotationSequence=XYX  RotationSequenceAngles=[0 0 0]  RotationSequenceAnglesUnits=deg  RotationMatrix=[1 0 0; 0 1 0; 0 0 1]
  h_39_axle_1_RIGID : Subsystem
      mask Display: image('h_39_axle_1_RIGID.JPG')
  h_axle_asymmetric_1_RIGID : Subsystem
      mask Display: image('h_axle_asymmetric_1_RIGID.JPG')
  h_collar_1_RIGID : Subsystem
      mask Display: image('h_collar_1_RIGID.JPG')
  h_connector_straight_1_RIGID : Subsystem
      mask Display: image('h_connector_straight_1_RIGID.JPG')
  B : PMIOPort  Side=Left
  F : PMIOPort  Port=2  Side=Right
  connections:
  Transform/LConn1 -- Transform1/LConn1 -- Transform2/LConn1 -- Transform3/LConn1 -- Transform4/LConn1 -- Transform5/LConn1
  Transform1/RConn1 -- F/RConn1
  Transform2/RConn1 -- h_axle_asymmetric_1_RIGID/LConn1
  Transform3/RConn1 -- h_connector_straight_1_RIGID/LConn1
  Transform4/RConn1 -- h_39_axle_1_RIGID/LConn1
  Transform5/RConn1 -- h_collar_1_RIGID/LConn1
  Transform/RConn1 -- B/RConn1
